simulink model "e_noisev1plusv2"  (R2021a)
settings: Solver=ode1  StartTime=0.0  StopTime=10.0  FixedStep=integration_step_size  RelTol=1e-3
values from neighbouring files (symbols this model uses):
  Gpert1s = Kpert1/(tal_pert1*s + 1)    [list1.m]
  Gpert2s = Kpert1/((tal_pert21*s + 1)*(tal_pert22*s + 1))    [list1.m]
  Gs = tf(K,[tal 1],'InputDelay',theta)    [list1.m]
libraries: commchan3 x4
settings Model: Creator=Fernando  LastModifiedBy=Fernando

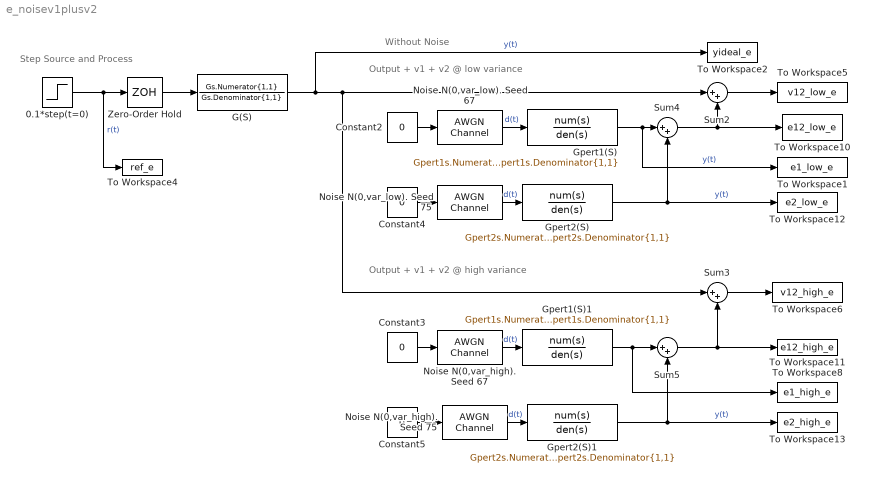
== system e_noisev1plusv2 ==
  note: Output + v1 + v2 @ high variance
  note: Output + v1 + v2 @ low variance
  note: Step Source and Process
  note: Without Noise
  0.1*step(t=0) : Step  Time=0  After=0.1  SampleTime=0
  Constant{2..5} (4 alike) : Constant  Value=0
  G(S) : TransferFcn  Numerator=Gs.Numerator{1,1}  Denominator=Gs.Denominator{1,1}
  Gpert1(S) : TransferFcn  Numerator=Gpert1s.Numerator{1,1}  Denominator=Gpert1s.Denominator{1,1}
  Gpert1(S)1 : TransferFcn  Numerator=Gpert1s.Numerator{1,1}  Denominator=Gpert1s.Denominator{1,1}
  Gpert2(S) : TransferFcn  Numerator=Gpert2s.Numerator{1,1}  Denominator=Gpert2s.Denominator{1,1}
  Gpert2(S)1 : TransferFcn  Numerator=Gpert2s.Numerator{1,1}  Denominator=Gpert2s.Denominator{1,1}
  Noise N(0,var_high). Seed 67 : commchan3/AWGN Channel  InputProcessing=Columns as channels (frame based)  seed=67  noiseMode=Variance from mask  EbNodB=10  EsNodB=10  SNRdB=10  bitsPerSym=1  Ps=1  Tsym=1  variance=var_high
  Noise N(0,var_high). Seed 75 : commchan3/AWGN Channel  InputProcessing=Columns as channels (frame based)  seed=75  noiseMode=Variance from mask  EbNodB=10  EsNodB=10  SNRdB=10  bitsPerSym=1  Ps=1  Tsym=1  variance=var_high
  Noise N(0,var_low). Seed 67 : commchan3/AWGN Channel  InputProcessing=Columns as channels (frame based)  seed=67  noiseMode=Variance from mask  EbNodB=10  EsNodB=10  SNRdB=10  bitsPerSym=1  Ps=1  Tsym=1  variance=var_low
  Noise N(0,var_low). Seed 75 : commchan3/AWGN Channel  InputProcessing=Columns as channels (frame based)  seed=75  noiseMode=Variance from mask  EbNodB=10  EsNodB=10  SNRdB=10  bitsPerSym=1  Ps=1  Tsym=1  variance=var_low
  Sum{2..5} (4 alike) : Sum  Inputs=|++
  To Workspace1 : ToWorkspace  VariableName=e1_low_e  SaveFormat=Timeseries  SampleTime=-1
      settings: Decimation=100
  To Workspace10 : ToWorkspace  VariableName=e12_low_e  SaveFormat=Timeseries  SampleTime=-1
      settings: Decimation=100
  To Workspace11 : ToWorkspace  VariableName=e12_high_e  SaveFormat=Timeseries  SampleTime=-1
      settings: Decimation=100
  To Workspace12 : ToWorkspace  VariableName=e2_low_e  SaveFormat=Timeseries  SampleTime=-1
      settings: Decimation=100
  To Workspace13 : ToWorkspace  VariableName=e2_high_e  SaveFormat=Timeseries  SampleTime=-1
      settings: Decimation=100
  To Workspace2 : ToWorkspace  VariableName=yideal_e  SaveFormat=Timeseries  SampleTime=-1
      settings: Decimation=100
  To Workspace4 : ToWorkspace  VariableName=ref_e  SaveFormat=Timeseries  SampleTime=-1
      settings: Decimation=100
  To Workspace5 : ToWorkspace  VariableName=v12_low_e  SaveFormat=Timeseries  SampleTime=-1
      settings: Decimation=100
  To Workspace6 : ToWorkspace  VariableName=v12_high_e  SaveFormat=Timeseries  SampleTime=-1
      settings: Decimation=100
  To Workspace8 : ToWorkspace  VariableName=e1_high_e  SaveFormat=Timeseries  SampleTime=-1
      settings: Decimation=100
  Zero-Order Hold : ZeroOrderHold  SampleTime=-1
  wires:
  G(S)/1 -> To Workspace2/1, Sum3/1, Sum2/1  "y(t)"
  Constant4/1 -> Noise N(0,var_low). Seed 75/1
  Gpert2(S)1/1 -> To Workspace13/1, Sum5/2  "y(t)"
  Gpert2(S)/1 -> Sum4/2, To Workspace12/1  "y(t)"
  Noise N(0,var_high). Seed 67/1 -> Gpert1(S)1/1  "d(t)"
  Noise N(0,var_low). Seed 75/1 -> Gpert2(S)/1  "d(t)"
  Sum3/1 -> To Workspace6/1
  0.1*step(t=0)/1 -> Zero-Order Hold/1, To Workspace4/1  "r(t)"
  Zero-Order Hold/1 -> G(S)/1
  Noise N(0,var_low). Seed 67/1 -> Gpert1(S)/1  "d(t)"
  Sum2/1 -> To Workspace5/1
  Constant2/1 -> Noise N(0,var_low). Seed 67/1
  Constant5/1 -> Noise N(0,var_high). Seed 75/1
  Noise N(0,var_high). Seed 75/1 -> Gpert2(S)1/1  "d(t)"
  Constant3/1 -> Noise N(0,var_high). Seed 67/1
  Sum4/1 -> Sum2/2, To Workspace10/1
  Gpert1(S)/1 -> To Workspace1/1, Sum4/1  "y(t)"
  Sum5/1 -> Sum3/2, To Workspace11/1
  Gpert1(S)1/1 -> To Workspace8/1, Sum5/1
